simulink model "PIL_NO_RPI"  (R2021a)
settings: Solver=FixedStepAuto  StartTime=0.0  StopTime=50  FixedStep=0.001  RelTol=1e-3  EnableMultiTasking=on
undefined symbols (not defined in the file or in its folder): act_dmp, act_omega, Actuator, Aerodynamics, aMode, Autopilot, c_b_WGS, c_be, c_flat, c_grav, c_h_geop0, c_h_geope, c_pa0, c_pe, c_r0, c_rot, c_rsma, c_Tmp0, d_siB_0, d_siB_max, d_siB_min, dd_siB_max, dd_siB_min, DiscIntNeverNeededParam, e_pa, e_Tmp, fin_maxrate, flag_I_act_switch, flag_I_aero_switch, flag_I_flat, flag_I_gravity_switch, flag_I_rot, hcr, HIL_Data, JMMM_0, JMMM_e, JSPB_e, lat_0, lon_0, Mass_Props, mB_0, mM_0, mM_e, p, pBII_0, phi, pMPB, pNPB, propellant_kg, prp_FBPB, prp_mdot, prp_T, psi, pSPB, q, qEG_0, qIB_0, qIE_0, r, sgc ... (+28)
libraries: simulink x46, simulink_extras x10, aerolibcommonsys x4
(part 5 of 21)

== system PIL_NO_RPI/Non-linear Flight Dynamic Model1/Subsystem1/GRM_Airframe/rb_eom ==
  mot_kin : Inport
  for_mom : Inport  Port=2
  wab : Inport  Port=3
  Bus Creator : BusCreator  Inputs=16
  calc_bus_flight_dyn_bus_entries : Subsystem
  eom_6dof : Subsystem
  flight_dyn : Outport  VectorParamsAs1DForOutWhenUnconnected=off
  wires:
  mot_kin/1 -> calc_bus_flight_dyn_bus_entries/1(mot_kin)
  calc_bus_flight_dyn_bus_entries/1(aBIB) -> Bus Creator/1
  calc_bus_flight_dyn_bus_entries/2(lon) -> Bus Creator/2
  calc_bus_flight_dyn_bus_entries/3(lat) -> Bus Creator/3
  calc_bus_flight_dyn_bus_entries/4(hBE) -> Bus Creator/4
  calc_bus_flight_dyn_bus_entries/5(vBII) -> Bus Creator/5
  calc_bus_flight_dyn_bus_entries/6(qIB) -> Bus Creator/6
  calc_bus_flight_dyn_bus_entries/7(wBIB) -> Bus Creator/7
  calc_bus_flight_dyn_bus_entries/8(d_wBIB) -> Bus Creator/8
  calc_bus_flight_dyn_bus_entries/9(d_vBII) -> Bus Creator/9
  Bus Creator/1 -> flight_dyn/1  "flight_dyn_bus"
  for_mom/1 -> eom_6dof/1(for_mom)
  wab/1 -> eom_6dof/2(wab)
  eom_6dof/1(eom) -> calc_bus_flight_dyn_bus_entries/2(eom)
  calc_bus_flight_dyn_bus_entries/10(pBII) -> Bus Creator/10
  calc_bus_flight_dyn_bus_entries/11(euIB) -> Bus Creator/11
  calc_bus_flight_dyn_bus_entries/12(vBIB) -> Bus Creator/12
  calc_bus_flight_dyn_bus_entries/13(qGB) -> Bus Creator/13
  calc_bus_flight_dyn_bus_entries/14(euGB) -> Bus Creator/14
  calc_bus_flight_dyn_bus_entries/15(euBG) -> Bus Creator/15
  calc_bus_flight_dyn_bus_entries/16(pBLG) -> Bus Creator/16

== system PIL_NO_RPI/Non-linear Flight Dynamic Model1/Subsystem1/GRM_Airframe/stream_flow ==
  flight_dyn : Inport
  motion_kin : Inport  Port=2
  env : Inport  Port=3
  Bus Selector1 : BusSelector  OutputSignals=atm_bus.atm_stat_bus.rho,atm_bus.atm_stat_bus.sos,atm_bus.atm_stat_bus.hBE
  Bus Selector2 : BusSelector  OutputSignals=vBII,pBII,wBIB
  Bus Selector3 : BusSelector  OutputSignals=TIB,wIEE,TIE
  calc_stream_flow : Subsystem
  str_flow : Outport  VectorParamsAs1DForOutWhenUnconnected=off
  wires:
  motion_kin/1 -> Bus Selector3/1
  flight_dyn/1 -> Bus Selector2/1
  env/1 -> Bus Selector1/1
  Bus Selector3/1 -> calc_stream_flow/1(TIB)  "<TIB>"
  Bus Selector3/2 -> calc_stream_flow/2(wIEE)  "<wIEE>"
  Bus Selector3/3 -> calc_stream_flow/3(TIE)  "<TIE>"
  Bus Selector2/1 -> calc_stream_flow/4(VBII)  "<vBII>"
  Bus Selector2/3 -> calc_stream_flow/6(wBIB)  "<wBIB>"
  Bus Selector1/1 -> calc_stream_flow/7(rho)  "<rho>"
  Bus Selector1/2 -> calc_stream_flow/8(sos)  "<sos>"
  Bus Selector1/3 -> calc_stream_flow/9(hBE)  "<hBE>"
  calc_stream_flow/1(str_flow) -> str_flow/1
  Bus Selector2/2 -> calc_stream_flow/5(pBII)  "<pBII>"

== system PIL_NO_RPI/Non-linear Flight Dynamic Model1/Subsystem1/GRM_Airframe/weight_and_balance ==
  env_glb : Inport
  Bus Creator1 : BusCreator  Inputs=3
  Bus Selector2 : BusSelector  OutputSignals=T_sim_glbl,T_sim_lnch
  Subtract : Sum  Inputs=+-
  center_of_gravity : Subsystem
  mass : Subsystem
  mass_uncertainty : Subsystem
  moi : Subsystem
  wab : Outport  VectorParamsAs1DForOutWhenUnconnected=off
  wires:
  Bus Selector2/2 -> Subtract/2  "<T_sim_lnch>"
  Bus Selector2/1 -> Subtract/1  "<T_sim_glbl>"
  env_glb/1 -> Bus Selector2/1
  Bus Creator1/1 -> wab/1  "wab_bus"
  center_of_gravity/1(pBPB) -> moi/1(pBPB), Bus Creator1/2
  moi/1(JBBB) -> Bus Creator1/3
  mass/2(mM) -> moi/2(mM), center_of_gravity/2(mM)
  mass_uncertainty/1(mB) -> center_of_gravity/1(mB), Bus Creator1/1
  mass/1(mB_c) -> mass_uncertainty/1(mB_c)
  Subtract/1 -> mass/1(sim_time_launch)

== system PIL_NO_RPI/Non-linear Flight Dynamic Model2/Extract Relevant States/Assemble_States_Bus1/Rotation Angles to Quaternions ==
  "R1, R2, R3" : Inport  Unit=rad
  1/2 : Gain  Gain=0.5  SaturateOnIntegerOverflow=on  OutDataTypeStr=Inherit: Same as input  ParamDataTypeStr=Inherit: Same as input
  Mux1 : Mux  Inputs=2
  Mux2 : Mux
  q0 : Fcn  Expr=u(4)*u(5)*u(6) + u(1)*u(2)*u(3)
  q1 : Fcn  Expr=u(4)*u(5)*u(3) - u(1)*u(2)*u(6)
  q2 : Fcn  Expr=u(4)*u(2)*u(6) + u(1)*u(5)*u(3)
  q3 : Fcn  Expr=u(1)*u(5)*u(6) - u(4)*u(2)*u(3)
  sincos : Trigonometry  Operator=sincos
  Quat : Outport  Unit=1  InitialOutput=0  VectorParamsAs1DForOutWhenUnconnected=off
  wires:
  q0/1 -> Mux2/1
  Mux2/1 -> Quat/1
  q3/1 -> Mux2/4
  q2/1 -> Mux2/3
  q1/1 -> Mux2/2
  Mux1/1 -> q3/1, q2/1, q1/1, q0/1
  sincos/2 -> Mux1/2
  sincos/1 -> Mux1/1
  1/2/1 -> sincos/1
  "R1, R2, R3"/1 -> 1/2/1

== system PIL_NO_RPI/Non-linear Flight Dynamic Model2/GRM_Airframe/aerodynamics/aerodynamic_via_lookup ==
  pBPB : Inport
  qdynB : Inport  Port=2
  MaB : Inport  Port=3
  alB : Inport  Port=4
  beB : Inport  Port=5
  hBE : Inport  Port=6
  wBIB_star : Inport  Port=7
  afinB : Inport  Port=8
  flag_I_prp : Inport  Port=9
  Bus Creator : BusCreator  Inputs=2
  Demux1 : Demux  Outputs=3
  Demux3 : Demux  Outputs=3
  Gain{,1..4} (5 alike) : Gain  Gain=180/pi
      settings: AttributesFormatString=%<Gain>
  Saturation1 : Saturate  UpperLimit=Aerodynamics.ulim_alpha_deg  LowerLimit=Aerodynamics.llim_alpha_deg
      settings: AttributesFormatString=|
      | %<UpperLimit>
      | %<LowerLimit>
  Saturation4 : Saturate  UpperLimit=Aerodynamics.ulim_beta_deg  LowerLimit=Aerodynamics.llim_beta_deg
      settings: AttributesFormatString=|
      | %<UpperLimit>
      | %<LowerLimit>
  Terminator : Terminator
  Terminator1 : Terminator
  calc_aero_coefficients : Subsystem
  calc_aero_for_mom : Subsystem
  aero_bus : Outport  VectorParamsAs1DForOutWhenUnconnected=off
  wires:
  Gain4/1 -> Saturation4/1
  Gain3/1 -> Saturation1/1
  Saturation4/1 -> calc_aero_coefficients/8(beB_deg)
  Saturation1/1 -> calc_aero_coefficients/7(alB_deg)
  calc_aero_coefficients/6(Cn) -> calc_aero_for_mom/9(Cn)
  calc_aero_coefficients/5(Cm) -> calc_aero_for_mom/8(Cm)
  calc_aero_coefficients/4(Cl) -> calc_aero_for_mom/7(Cl)
  calc_aero_coefficients/3(Cz) -> calc_aero_for_mom/6(Cz)
  calc_aero_coefficients/2(Cy) -> calc_aero_for_mom/5(Cy)
  calc_aero_coefficients/1(Cx) -> calc_aero_for_mom/4(Cx)
  Gain2/1 -> calc_aero_coefficients/3(delr_deg)
  Gain1/1 -> calc_aero_coefficients/2(dele_deg)
  Gain/1 -> calc_aero_coefficients/1(dela_deg)
  Demux3/3 -> Gain2/1  "zeB"
  Demux3/1 -> Gain/1  "xiB"
  Demux3/2 -> Gain1/1  "etB"
  afinB/1 -> Demux3/1
  Demux1/3 -> calc_aero_coefficients/6(rBIB_star_rps)  "rBIB_star_rps"
  Demux1/2 -> calc_aero_coefficients/5(qBIB_star_rps)  "qBIB_star_rps"
  Demux1/1 -> calc_aero_coefficients/4(pBIB_star_rps)  "pBIB_star_rps"
  wBIB_star/1 -> Demux1/1
  beB/1 -> Gain4/1
  alB/1 -> Gain3/1
  qdynB/1 -> calc_aero_for_mom/3(qdynB)
  calc_aero_for_mom/2(MBAB) -> Bus Creator/2
  hBE/1 -> calc_aero_for_mom/1(hBE)
  flag_I_prp/1 -> Terminator/1
  pBPB/1 -> calc_aero_for_mom/2(pBPB)
  Bus Creator/1 -> aero_bus/1  "aero_bus"
  calc_aero_for_mom/1(FBAB) -> Bus Creator/1
  MaB/1 -> Terminator1/1

== system PIL_NO_RPI/Non-linear Flight Dynamic Model2/GRM_Airframe/aerodynamics/logic_base_drag ==
  env_glbl : Inport
  Bus Selector1 : BusSelector  OutputSignals=T_sim_glbl,T_sim_lnch
  Constant : Constant  Value=prp_T(end)
  MATLAB Function : MATLAB Function  TreatAsAtomicUnit=on
  Subtract : Sum  Inputs=+-
  flag_base_drag : Outport  VectorParamsAs1DForOutWhenUnconnected=off
  wires:
  env_glbl/1 -> Bus Selector1/1
  Bus Selector1/2 -> Subtract/2  "<T_sim_lnch>"
  Bus Selector1/1 -> Subtract/1  "<T_sim_glbl>"
  MATLAB Function/1(flag_base_drag) -> flag_base_drag/1  "flag_base_drag"
  Constant/1 -> MATLAB Function/2(t_prp2)
  Subtract/1 -> MATLAB Function/1(u)

== system PIL_NO_RPI/Non-linear Flight Dynamic Model2/GRM_Airframe/environment/WGS84_Gravitation ==
  lon : Inport  PortDimensions=1
  lat : Inport  Port=2  PortDimensions=1
  h : Inport  Port=3  PortDimensions=1
  Assertion : Assertion  AssertionFailFcn="error('WGS84 Gravitationsmodell: Die Werte des Eingangs \"h\" muessen groesser als 0 sein')"
  Assertion1 : Assertion  AssertionFailFcn="error('WGS84 Gravitationsmodell: Die Werte des Eingangs \"Long\" muessen zwischen -180 und +180 liegen')"
  Assertion2 : Assertion  AssertionFailFcn="error('WGS84 Gravitationsmodell: Die Werte des Eingangs \"Lat\" muessen zwischen -90 und +90 liegen')"
  Compare To Constant : simulink/Logic and Bit Operations/Compare To Constant  relop=>=  const=0  OutDataTypeStr=boolean
      settings: SourceProductName=ISim Simulink Block Set
  Interval Test : simulink/Logic and Bit Operations/Interval Test  IntervalClosedRight=on  uplimit=pi  IntervalClosedLeft=on  lowlimit=-pi  OutDataTypeStr=boolean
      settings: SourceProductName=ISim Simulink Block Set
  Interval Test1 : simulink/Logic and Bit Operations/Interval Test  IntervalClosedRight=on  uplimit=pi/2  IntervalClosedLeft=on  lowlimit=-pi/2  OutDataTypeStr=boolean
      settings: SourceProductName=ISim Simulink Block Set
  WGS84_2_ECEF : Subsystem
  WGS84_Gravity_Implementation : MATLAB Function  TreatAsAtomicUnit=on
  gE : Outport  PortDimensions=3  VectorParamsAs1DForOutWhenUnconnected=off
  wires:
  WGS84_Gravity_Implementation/1(gamma_R) -> gE/1  "gE"
  h/1 -> Compare To Constant/1, WGS84_2_ECEF/1(h)  "h"
  lon/1 -> WGS84_2_ECEF/2(lon), Interval Test/1, WGS84_Gravity_Implementation/3(long_rad)  "lon"
  lat/1 -> WGS84_2_ECEF/3(lat), Interval Test1/1, WGS84_Gravity_Implementation/2(lat_rad)  "lat"
  WGS84_2_ECEF/1(pE) -> WGS84_Gravity_Implementation/1(pE)  "pE"
  Compare To Constant/1 -> Assertion/1
  Interval Test/1 -> Assertion1/1
  Interval Test1/1 -> Assertion2/1

== system PIL_NO_RPI/Non-linear Flight Dynamic Model2/GRM_Airframe/environment/atmosphere_static_ISO_2533 ==
  hBE : Inport
  env_glbl : Inport  Port=2
  Bus Creator1 : BusCreator  Inputs=6
  Bus Selector1 : BusSelector  OutputSignals=e_Tmp,e_pa
  Saturation : Saturate  UpperLimit=c_h_geope  LowerLimit=c_h_geop0
      settings: AttributesFormatString=|
      | %<UpperLimit>
      | %<LowerLimit>
  density : Subsystem
  geopot_height : Subsystem  mask{mean_earth_radius=c_r0}
      mask prompts: mean_earth_radius "Mean Earth Radius WGS 84 [m]"
      mask TypeOptions mean_earth_radius: mean_earth_radius/Value
  speed_of_sound : Subsystem
  tmp_and_pressure_ISO_2533 : Subsystem
  atm_stat : Outport  VectorParamsAs1DForOutWhenUnconnected=off
  wires:
  Saturation/1 -> tmp_and_pressure_ISO_2533/1(h_geop), Bus Creator1/2  "h_geop"
  hBE/1 -> geopot_height/1(hBE), Bus Creator1/1
  density/1(rho) -> Bus Creator1/5
  tmp_and_pressure_ISO_2533/2(pa) -> density/2(pa), Bus Creator1/6
  tmp_and_pressure_ISO_2533/1(Tmp) -> density/1(Tmp), Bus Creator1/4, speed_of_sound/1(Tmp)
  Bus Creator1/1 -> atm_stat/1  "atm_stat_bus"
  Bus Selector1/1 -> tmp_and_pressure_ISO_2533/2(e_Tmp)  "<e_Tmp>"
  geopot_height/1(h_geop) -> Saturation/1
  Bus Selector1/2 -> tmp_and_pressure_ISO_2533/3(e_pa)  "<e_pa>"
  env_glbl/1 -> Bus Selector1/1
  speed_of_sound/1(sos) -> Bus Creator1/3

== system PIL_NO_RPI/Non-linear Flight Dynamic Model2/GRM_Airframe/environment/convert_to_local_frame ==
  gE : Inport
  Constant1 : Constant  Value=0
  Dot Product : DotProduct  InputSameDT=on  OutDataTypeStr=Inherit: Inherit via internal rule
  Sqrt : Sqrt  SaturateOnIntegerOverflow=on
  Vector Concatenate : Concatenate  NumInputs=3  Mode=Multidimensional array
  gBG : Outport  VectorParamsAs1DForOutWhenUnconnected=off
  wires:
  Dot Product/1 -> Sqrt/1
  Vector Concatenate/1 -> gBG/1  "gBG"
  Sqrt/1 -> Vector Concatenate/3
  Constant1/1 -> Vector Concatenate/1, Vector Concatenate/2
  gE/1 -> Dot Product/2, Dot Product/1

== system PIL_NO_RPI/Non-linear Flight Dynamic Model2/GRM_Airframe/fin_actuators/Rudder ==
  siB_c : Inport
  tRRR : Inport  Port=2
  Add : Sum  Inputs=+-
  Add1 : Sum  Inputs=+-
  Add2 : Sum  Inputs=+++
  Constant1 : Constant  Value=Actuator.fin1_bias
      settings: AttributesFormatString=%<Value>
  Gain : Gain  Gain=omega^2
  Gain2 : Gain  Gain=2*dmp*omega  Multiplication=Matrix(K*u)
  Gain3 : Gain  Gain=unc_bl
  Gain4 : Gain  Gain=Actuator.fin1_scale
      settings: AttributesFormatString=%<Gain>
  Integrator : Integrator  ExternalReset=either  InitialCondition=d_siB_0
  Integrator1 : Integrator  InitialCondition=siB_0  LimitOutput=on  UpperSaturationLimit=siB_max  LowerSaturationLimit=siB_min  ShowSaturationPort=on
  Limiting_Acceleration : MATLAB Function  TreatAsAtomicUnit=on
  Limiting_Rate : MATLAB Function  TreatAsAtomicUnit=on
  Saturation : Saturate  UpperLimit=siB_max  LowerLimit=siB_min
  Saturation1 : Saturate  UpperLimit=siB_max  LowerLimit=siB_min
  Sign : Signum
  siB : Outport  VectorParamsAs1DForOutWhenUnconnected=off
  d_siB : Outport  Port=2  VectorParamsAs1DForOutWhenUnconnected=off
  dd_siB : Outport  Port=3  VectorParamsAs1DForOutWhenUnconnected=off
  wires:
  [siB] -> Limiting_Rate/1(siB)
  [siB] -> Limiting_Acceleration/1(siB)
  [d_siB] -> Limiting_Acceleration/2(d_siB)
  siB_c/1 -> Saturation/1  "siB_c"
  Constant1/1 -> Add2/1
  Add2/1 -> Saturation1/1
  Saturation/1 -> Add/1
  Integrator/1 -> Gain2/1, Limiting_Rate/2(d_siB)  "d_siB"
  Limiting_Rate/1(d_siB_l) -> Integrator1/1, [d_siB], d_siB/1  "d_siB_l"
  Limiting_Acceleration/1(dd_siB_l) -> dd_siB/1, Integrator/1  "dd_siB_l"
  Add/1 -> Gain/1
  Gain/1 -> Add1/1
  Gain2/1 -> Add1/2
  Add1/1 -> Limiting_Acceleration/3(dd_siB)  "dd_siB"
  Integrator1/1 -> Add/2, Gain4/1  "siB"
  tRRR/1 -> Sign/1  "tRRR"
  Sign/1 -> Gain3/1
  Gain3/1 -> Add2/3
  Gain4/1 -> Add2/2
  Integrator1/2 -> Integrator/2  "sat"
  Saturation1/1 -> [siB], siB/1  "siB"

== system PIL_NO_RPI/Non-linear Flight Dynamic Model2/GRM_Airframe/fin_actuators/Rudder1 ==
  siB_c : Inport
  tRRR : Inport  Port=2
  Add : Sum  Inputs=+-
  Add1 : Sum  Inputs=+-
  Add3 : Sum  Inputs=+++
  Constant1 : Constant  Value=Actuator.fin2_bias
      settings: AttributesFormatString=%<Value>
  Gain : Gain  Gain=omega^2
  Gain2 : Gain  Gain=2*dmp*omega  Multiplication=Matrix(K*u)
  Gain3 : Gain  Gain=unc_bl
  Gain4 : Gain  Gain=Actuator.fin2_scale
      settings: AttributesFormatString=%<Gain>
  Integrator : Integrator  ExternalReset=either  InitialCondition=d_siB_0
  Integrator1 : Integrator  InitialCondition=siB_0  LimitOutput=on  UpperSaturationLimit=siB_max  LowerSaturationLimit=siB_min  ShowSaturationPort=on
  Limiting_Acceleration : MATLAB Function  TreatAsAtomicUnit=on
  Limiting_Rate : MATLAB Function  TreatAsAtomicUnit=on
  Saturation : Saturate  UpperLimit=siB_max  LowerLimit=siB_min
  Saturation1 : Saturate  UpperLimit=siB_max  LowerLimit=siB_min
  Sign : Signum
  siB : Outport  VectorParamsAs1DForOutWhenUnconnected=off
  d_siB : Outport  Port=2  VectorParamsAs1DForOutWhenUnconnected=off
  dd_siB : Outport  Port=3  VectorParamsAs1DForOutWhenUnconnected=off
  wires:
  Gain4/1 -> Add3/2
  Constant1/1 -> Add3/1
  [siB] -> Limiting_Rate/1(siB)
  [siB] -> Limiting_Acceleration/1(siB)
  [d_siB] -> Limiting_Acceleration/2(d_siB)
  siB_c/1 -> Saturation/1  "siB_c"
  Add3/1 -> Saturation1/1
  Saturation/1 -> Add/1
  Integrator/1 -> Gain2/1, Limiting_Rate/2(d_siB)  "d_siB"
  Limiting_Rate/1(d_siB_l) -> Integrator1/1, [d_siB], d_siB/1  "d_siB_l"
  Limiting_Acceleration/1(dd_siB_l) -> dd_siB/1, Integrator/1  "dd_siB_l"
  Add/1 -> Gain/1
  Gain/1 -> Add1/1
  Gain2/1 -> Add1/2
  Add1/1 -> Limiting_Acceleration/3(dd_siB)  "dd_siB"
  Integrator1/1 -> Gain4/1, Add/2  "siB"
  tRRR/1 -> Sign/1  "tRRR"
  Sign/1 -> Gain3/1
  Gain3/1 -> Add3/3
  Integrator1/2 -> Integrator/2  "sat"
  Saturation1/1 -> [siB], siB/1  "siB"

== system PIL_NO_RPI/Non-linear Flight Dynamic Model2/GRM_Airframe/fin_actuators/Rudder2 ==
  siB_c : Inport
  tRRR : Inport  Port=2
  Add : Sum  Inputs=+-
  Add1 : Sum  Inputs=+-
  Add3 : Sum  Inputs=+++
  Constant1 : Constant  Value=Actuator.fin3_bias
      settings: AttributesFormatString=%<Value>
  Gain : Gain  Gain=omega^2
  Gain2 : Gain  Gain=2*dmp*omega  Multiplication=Matrix(K*u)
  Gain3 : Gain  Gain=unc_bl
  Gain4 : Gain  Gain=Actuator.fin3_scale
      settings: AttributesFormatString=%<Gain>
  Integrator : Integrator  ExternalReset=either  InitialCondition=d_siB_0
  Integrator1 : Integrator  InitialCondition=siB_0  LimitOutput=on  UpperSaturationLimit=siB_max  LowerSaturationLimit=siB_min  ShowSaturationPort=on
  Limiting_Acceleration : MATLAB Function  TreatAsAtomicUnit=on
  Limiting_Rate : MATLAB Function  TreatAsAtomicUnit=on
  Saturation : Saturate  UpperLimit=siB_max  LowerLimit=siB_min
  Saturation1 : Saturate  UpperLimit=siB_max  LowerLimit=siB_min
  Sign : Signum
  siB : Outport  VectorParamsAs1DForOutWhenUnconnected=off
  d_siB : Outport  Port=2  VectorParamsAs1DForOutWhenUnconnected=off
  dd_siB : Outport  Port=3  VectorParamsAs1DForOutWhenUnconnected=off
  wires:
  Gain4/1 -> Add3/2
  Constant1/1 -> Add3/1
  [siB] -> Limiting_Rate/1(siB)
  [siB] -> Limiting_Acceleration/1(siB)
  [d_siB] -> Limiting_Acceleration/2(d_siB)
  siB_c/1 -> Saturation/1  "siB_c"
  Add3/1 -> Saturation1/1
  Saturation/1 -> Add/1
  Integrator/1 -> Gain2/1, Limiting_Rate/2(d_siB)  "d_siB"
  Limiting_Rate/1(d_siB_l) -> Integrator1/1, [d_siB], d_siB/1  "d_siB_l"
  Limiting_Acceleration/1(dd_siB_l) -> dd_siB/1, Integrator/1  "dd_siB_l"
  Add/1 -> Gain/1
  Gain/1 -> Add1/1
  Gain2/1 -> Add1/2
  Add1/1 -> Limiting_Acceleration/3(dd_siB)  "dd_siB"
  Integrator1/1 -> Add/2, Gain4/1  "siB"
  tRRR/1 -> Sign/1  "tRRR"
  Sign/1 -> Gain3/1
  Gain3/1 -> Add3/3
  Integrator1/2 -> Integrator/2  "sat"
  Saturation1/1 -> [siB], siB/1  "siB"

== system PIL_NO_RPI/Non-linear Flight Dynamic Model2/GRM_Airframe/fin_actuators/Rudder3 ==
  siB_c : Inport
  tRRR : Inport  Port=2
  Add : Sum  Inputs=+-
  Add1 : Sum  Inputs=+-
  Add3 : Sum  Inputs=+++
  Constant1 : Constant  Value=Actuator.fin4_bias
      settings: AttributesFormatString=%<Value>
  Gain : Gain  Gain=omega^2
  Gain2 : Gain  Gain=2*dmp*omega  Multiplication=Matrix(K*u)
  Gain3 : Gain  Gain=unc_bl
  Gain4 : Gain  Gain=Actuator.fin4_scale
      settings: AttributesFormatString=%<Gain>
  Integrator : Integrator  ExternalReset=either  InitialCondition=d_siB_0
  Integrator1 : Integrator  InitialCondition=siB_0  LimitOutput=on  UpperSaturationLimit=siB_max  LowerSaturationLimit=siB_min  ShowSaturationPort=on
  Limiting_Acceleration : MATLAB Function  TreatAsAtomicUnit=on
  Limiting_Rate : MATLAB Function  TreatAsAtomicUnit=on
  Saturation : Saturate  UpperLimit=siB_max  LowerLimit=siB_min
  Saturation1 : Saturate  UpperLimit=siB_max  LowerLimit=siB_min
  Sign : Signum
  siB : Outport  VectorParamsAs1DForOutWhenUnconnected=off
  d_siB : Outport  Port=2  VectorParamsAs1DForOutWhenUnconnected=off
  dd_siB : Outport  Port=3  VectorParamsAs1DForOutWhenUnconnected=off
  wires:
  Gain4/1 -> Add3/2
  Constant1/1 -> Add3/1
  [siB] -> Limiting_Rate/1(siB)
  [siB] -> Limiting_Acceleration/1(siB)
  [d_siB] -> Limiting_Acceleration/2(d_siB)
  siB_c/1 -> Saturation/1  "siB_c"
  Add3/1 -> Saturation1/1
  Saturation/1 -> Add/1
  Integrator/1 -> Gain2/1, Limiting_Rate/2(d_siB)  "d_siB"
  Limiting_Rate/1(d_siB_l) -> Integrator1/1, [d_siB], d_siB/1  "d_siB_l"
  Limiting_Acceleration/1(dd_siB_l) -> dd_siB/1, Integrator/1  "dd_siB_l"
  Add/1 -> Gain/1
  Gain/1 -> Add1/1
  Gain2/1 -> Add1/2
  Add1/1 -> Limiting_Acceleration/3(dd_siB)  "dd_siB"
  Integrator1/1 -> Add/2, Gain4/1  "siB"
  tRRR/1 -> Sign/1  "tRRR"
  Sign/1 -> Gain3/1
  Gain3/1 -> Add3/3
  Integrator1/2 -> Integrator/2  "sat"
  Saturation1/1 -> [siB], siB/1  "siB"

== system PIL_NO_RPI/Non-linear Flight Dynamic Model2/GRM_Airframe/fin_actuators/control_allocation ==
  siB : Inport
  d_siB : Inport  Port=2
  dd_siB : Inport  Port=3
  Constant8 : Constant  Value=Tr3r4
  Product : Product  Multiplication=Matrix(*)
  Product1 : Product  Multiplication=Matrix(*)
  Product2 : Product  Multiplication=Matrix(*)
  Tr3r4 : Outport  VectorParamsAs1DForOutWhenUnconnected=off
  finB : Outport  Port=2  VectorParamsAs1DForOutWhenUnconnected=off
  d_finB : Outport  Port=3  VectorParamsAs1DForOutWhenUnconnected=off
  dd_finB : Outport  Port=4  VectorParamsAs1DForOutWhenUnconnected=off
  wires:
  Product2/1 -> dd_finB/1  "dd_afinB"
  dd_siB/1 -> Product2/2
  Product1/1 -> d_finB/1  "d_afinB"
  d_siB/1 -> Product1/2
  siB/1 -> Product/2
  Constant8/1 -> Product/1, Product1/1, Product2/1, Tr3r4/1  "Tr3r4"
  Product/1 -> finB/1  "afinB"

== system PIL_NO_RPI/Non-linear Flight Dynamic Model2/GRM_Airframe/gravity/launch_rail ==
  gBG_c : Inport
  hBE : Inport  Port=2
  Constant1 : Constant  Value=flag_I_gravity_switch
  Constant3 : Constant  Value=0
  Subtract : Sum  Inputs=++-
  Switch : Switch  Criteria=u2 > Threshold  Threshold=0.05
  Vector Concatenate : Concatenate  NumInputs=3
  initial_altitude : Subsystem
  gBG : Outport  VectorParamsAs1DForOutWhenUnconnected=off
  wires:
  initial_altitude/1(hBE_0) -> Subtract/3
  gBG_c/1 -> Switch/1
  Vector Concatenate/1 -> Switch/3
  Switch/1 -> gBG/1  "gBG"
  Constant3/1 -> Vector Concatenate/3, Vector Concatenate/2, Vector Concatenate/1
  Subtract/1 -> Switch/2
  hBE/1 -> Subtract/1
  Constant1/1 -> Subtract/2

== system PIL_NO_RPI/Non-linear Flight Dynamic Model2/GRM_Airframe/motion_kinematics/calc_motion_kinematics ==
  lat : Inport
  lon : Inport  Port=2
  qIB : Inport  Port=3
  calc_transformation_matrix : Subsystem
  earth_rotation : Subsystem
  wIEE : Outport  VectorParamsAs1DForOutWhenUnconnected=off
  TIE : Outport  Port=2  VectorParamsAs1DForOutWhenUnconnected=off
  TEB : Outport  Port=3  VectorParamsAs1DForOutWhenUnconnected=off
  TGB : Outport  Port=4  VectorParamsAs1DForOutWhenUnconnected=off
  TEG : Outport  Port=5  VectorParamsAs1DForOutWhenUnconnected=off
  wEGG : Outport  Port=6  VectorParamsAs1DForOutWhenUnconnected=off
  TIB : Outport  Port=7  VectorParamsAs1DForOutWhenUnconnected=off
  wires:
  calc_transformation_matrix/3(TIB) -> TIB/1
  calc_transformation_matrix/2(TGB) -> TGB/1
  calc_transformation_matrix/1(TEB) -> TEB/1
  qIB/1 -> calc_transformation_matrix/3(qIB)
  earth_rotation/4(qEG) -> calc_transformation_matrix/2(qEG)
  earth_rotation/3(qIE) -> calc_transformation_matrix/1(qIE)
  lat/1 -> earth_rotation/1(lat)
  lon/1 -> earth_rotation/2(lon)
  earth_rotation/6(wEGG) -> wEGG/1
  earth_rotation/5(TEG) -> TEG/1
  earth_rotation/2(TIE) -> TIE/1
  earth_rotation/1(wIEE) -> wIEE/1

== system PIL_NO_RPI/Non-linear Flight Dynamic Model2/GRM_Airframe/propulsion/prp_look_up ==
  env_glbl_bus : Inport
  Bus Selector1 : BusSelector  OutputSignals=T_sim_glbl,T_sim_lnch
  Constant : Constant  Value=0
  Constant1 : Constant  Value=0
  Saturation : Saturate  UpperLimit=prp_T(end)  LowerLimit=0
      settings: AttributesFormatString=|
      | %<UpperLimit>
      | %<LowerLimit>
  Subtract : Sum  Inputs=+-
  Switch : Switch  Criteria=u2 > Threshold
  Switch1 : Switch  Criteria=u2 > Threshold
  Vector Concatenate : Concatenate  NumInputs=3
  thrust_lookup : Lookup_n-D  NumberOfTableDimensions=1  BreakpointsForDimension1=prp_T  Table=prp_FBPB  ExtrapMethod=Clip  UseLastTableValue=on  InternalRulePriority=Speed  RndMeth=Simplest  InputSameDT=on
  FBPM : Outport  VectorParamsAs1DForOutWhenUnconnected=off
  wires:
  Switch1/1 -> Vector Concatenate/1  "a_FBPM"
  Constant1/1 -> Vector Concatenate/2, Vector Concatenate/3
  Vector Concatenate/1 -> FBPM/1  "FBPM"
  Saturation/1 -> thrust_lookup/1
  Subtract/1 -> Switch/2, Switch/1
  Constant/1 -> Switch/3
  env_glbl_bus/1 -> Bus Selector1/1
  Bus Selector1/1 -> Subtract/1  "<T_sim_glbl>"
  thrust_lookup/1 -> Switch1/1
  Switch/1 -> Switch1/3, Switch1/2, Saturation/1
  Bus Selector1/2 -> Subtract/2  "<T_sim_lnch>"

== system PIL_NO_RPI/Non-linear Flight Dynamic Model2/GRM_Airframe/propulsion/prp_uncertainty ==
  FBPM : Inport
  wab : Inport  Port=2
  3_rot_mat : Subsystem  mask(Rotation um 1, 2 oder 3 Achsen){rot_1=Rotation um z-Achse, rot_2=Rotation um y-Achse, rot_3=Rotation um x-Achse}
      mask prompts: rot_1 "1. Rotation"; rot_2 "2. Rotation"; rot_3 "3. Rotation"
      mask help:
      | Dieser Block liefert die Rotationsmatrix T12 für den Fall zurück, dass sich das Ziel-Koordinatensystem (1) durch Drehungen um 1, 2 oder 3 Achsen gegenüber dem Ausgangskoordinatensystem (2) beschreiben lässt (passive Drehung).
      |
      | Die Anzahl der Rotation sowie die Reihenfolge ist frei einstellbar.
      |
      | Die Rotationswinkel haben die Einheit [rad].
      mask TypeOptions rot_1: Rotation um x-Achse | Rotation um y-Achse | Rotation um z-Achse
      mask TypeOptions rot_2: Rotation um x-Achse | Rotation um y-Achse | Rotation um z-Achse
      mask TypeOptions rot_3: Rotation um x-Achse | Rotation um y-Achse | Rotation um z-Achse
  Bus Selector : BusSelector  OutputSignals=pBPB
  Product : Product  Multiplication=Matrix(*)
  Product1 : Product
  Subtract : Sum  Inputs=+-
  Thrust_rot_z : Constant  Value=unc_prp_z
  cross_product : Subsystem
      mask help: cross product r3 = r1 x r2
      mask Help:
      | Name:
      | 
      |     cross_product
      | 
      | Description:
      | 
      |     This block implements the cross product r3 = r1 x r2.
      | 
      | Inputs  [size] [data type] [unit]:
      | 
      |     vector 1  [3] [double] [-]
      |     vector 2  [3] [double] [-]
      | 
      | Outputs  [size] [data type] [unit]:
      | 
      |     resulting vector  [3] [double] [-]
      mask Display: disp(' r3 = r1 x r2')
  pNPB : Constant  Value=pNPB
  thrust_rot_x : Constant  Value=unc_prp_x
  thrust_rot_y : Constant  Value=unc_prp_y
  uncert_thrust : Constant  Value=unc_prp_scale
  FBPB : Outport  VectorParamsAs1DForOutWhenUnconnected=off
  MBPB : Outport  Port=2  VectorParamsAs1DForOutWhenUnconnected=off
  wires:
  Subtract/1 -> cross_product/1(r1)
  pNPB/1 -> Subtract/2
  Product1/1 -> Product/2
  uncert_thrust/1 -> Product1/2
  Bus Selector/1 -> Subtract/1  "<pBPB>"
  wab/1 -> Bus Selector/1
  cross_product/1(r1_x_r2) -> MBPB/1  "MBPB"
  thrust_rot_y/1 -> 3_rot_mat/2(wi2)
  3_rot_mat/1(T12) -> Product/1
  FBPM/1 -> Product1/1
  Product/1 -> FBPB/1, cross_product/2(r2)  "FBPB"
  thrust_rot_x/1 -> 3_rot_mat/3(wi3)
  Thrust_rot_z/1 -> 3_rot_mat/1(wi1)

== system PIL_NO_RPI/Non-linear Flight Dynamic Model2/GRM_Airframe/rb_eom/calc_bus_flight_dyn_bus_entries ==
  mot_kin : Inport
  eom : Inport  Port=2
  Bus Selector : BusSelector  OutputSignals=pBII,vBII,qIB,wBIB,d_wBIB,d_vBII
  Bus Selector1 : BusSelector  OutputSignals=pBII
  Bus Selector3 : BusSelector  OutputSignals=TGB,TIB,TIE
  Constant : Constant  Value=pBII_0
      settings: AttributesFormatString=%<Value>
  Gain : Gain  Gain=-1
  Math Function : Math  Operator=transpose  SignedPower=on  SaturateOnIntegerOverflow=on
  Product{,1..3} (4 alike) : Product  Multiplication=Matrix(*)
  Subsystem2 : Subsystem
  Sum : Sum  Inputs=+-
  eom D1 : InportShadow  Port=2
  q12_from_T12 : Subsystem
      mask help: Transforms a Direction Cosine Matrix into a Quaternion
      mask Help:
      | Name:
      | 
      |     q12_from_T12
      | 
      | Description:
      | 
      |     This block implements the transformation of a direction cosine matrix DCM
      |      into the corresponding quaternion.
      | 
      | Inputs  [size] [data type] [unit]:
      | 
      |     direction cosine matrix T12  [3x3] [double] [-]
      | 
      | Outputs  [size] [data type] [unit]:
      | 
      |     quaternion q12  [4] [double] [-]
      mask Display:
      | %port_label('input', 1, 'T12')
      | %port_label('output', 1, 'q12')
      | disp('DCM \rightarrow q','texmode','on')
  quaternion_to_euler_angles : Subsystem
      mask help: transforms quaternions to Euler angles (roll, pitch, yaw)
      mask Help:
      | Name:
      | 
      |     quaternion_to_euler_angles
      | 
      | Description:
      | 
      |     This block implements the transformation of a quaternion into the
      |     corresponding Euler angles (zyx-sequence, roll, pitch, yaw).
      | 
      | Inputs  [size] [data type] [unit]:
      | 
      |     quaternion  [4] [double] [-]
      | 
      | Outputs  [size] [data type] [unit]:
      | 
      |     roll angle phi  [1] [double] [rad]
      |     pitch angle theta  [1] [double] [rad]
      |     yaw angle psi  [1] [double] [rad]
      mask Display:
      | %disp (' q --> (Phi,Theta,Psi) [rad]')
      | disp('q \rightarrow eu(\Phi;\Theta;\Psi)','texmode','on')
  quaternion_to_euler_angles1 : Subsystem
      mask help: transforms quaternions to Euler angles (roll, pitch, yaw)
      mask Help:
      | Name:
      | 
      |     quaternion_to_euler_angles
      | 
      | Description:
      | 
      |     This block implements the transformation of a quaternion into the
      |     corresponding Euler angles (zyx-sequence, roll, pitch, yaw).
      | 
      | Inputs  [size] [data type] [unit]:
      | 
      |     quaternion  [4] [double] [-]
      | 
      | Outputs  [size] [data type] [unit]:
      | 
      |     roll angle phi  [1] [double] [rad]
      |     pitch angle theta  [1] [double] [rad]
      |     yaw angle psi  [1] [double] [rad]
      mask Display:
      | %disp (' q --> (Phi,Theta,Psi) [rad]')
      | disp('q \rightarrow eu(\Phi;\Theta;\Psi)','texmode','on')
  aBIB : Outport  VectorParamsAs1DForOutWhenUnconnected=off
  lon : Outport  Port=2  VectorParamsAs1DForOutWhenUnconnected=off
  lat : Outport  Port=3  VectorParamsAs1DForOutWhenUnconnected=off
  hBE : Outport  Port=4  VectorParamsAs1DForOutWhenUnconnected=off
  vBII : Outport  Port=5  VectorParamsAs1DForOutWhenUnconnected=off
  qIB : Outport  Port=6  VectorParamsAs1DForOutWhenUnconnected=off
  wBIB : Outport  Port=7  VectorParamsAs1DForOutWhenUnconnected=off
  d_wBIB : Outport  Port=8  VectorParamsAs1DForOutWhenUnconnected=off
  d_vBII : Outport  Port=9  VectorParamsAs1DForOutWhenUnconnected=off
  pBII : Outport  Port=10  VectorParamsAs1DForOutWhenUnconnected=off
  euIB : Outport  Port=11  VectorParamsAs1DForOutWhenUnconnected=off
  vBIB : Outport  Port=12  VectorParamsAs1DForOutWhenUnconnected=off
  qGB : Outport  Port=13  VectorParamsAs1DForOutWhenUnconnected=off
  euGB : Outport  Port=14  VectorParamsAs1DForOutWhenUnconnected=off
  euBG : Outport  Port=15  VectorParamsAs1DForOutWhenUnconnected=off
  pBLG : Outport  Port=16  VectorParamsAs1DForOutWhenUnconnected=off
  wires:
  Product3/1 -> pBLG/1  "pBLG"
  Product2/1 -> Product3/1  "TGI"
  [TBI] -> Product2/2
  [TGB] -> Product2/1
  Sum/1 -> Product3/2  "pBLI"
  Constant/1 -> Sum/2
  Bus Selector1/1 -> Sum/1  "<pBII>"
  eom D1/1 -> Bus Selector1/1
  Gain/1 -> euBG/1  "euBG"
  quaternion_to_euler_angles1/1(eulx) -> Gain/1, euGB/1  "euGB"
  q12_from_T12/1(q12) -> qGB/1, quaternion_to_euler_angles1/1(q)  "qGB"
  Bus Selector3/1 -> q12_from_T12/1(T12), [TGB]  "<TGB>"
  Product1/1 -> vBIB/1  "vBIB"
  quaternion_to_euler_angles/1(eulx) -> euIB/1  "euIB"
  Bus Selector/5 -> d_wBIB/1  "<d_wBIB>"
  Bus Selector/4 -> wBIB/1  "<wBIB>"
  Bus Selector/3 -> qIB/1, quaternion_to_euler_angles/1(q)  "<qIB>"
  Bus Selector/2 -> vBII/1, Product1/2  "<vBII>"
  Subsystem2/3(hBE) -> hBE/1  "hBE"
  Subsystem2/2(lat) -> lat/1
  Subsystem2/1(lon) -> lon/1
  Product/1 -> aBIB/1  "aBIB"
  Bus Selector/6 -> d_vBII/1, Product/2  "<d_vBII>"
  Bus Selector3/2 -> Math Function/1  "<TIB>"
  Math Function/1 -> Product/1, Product1/1, [TBI]  "TBI"
  eom/1 -> Bus Selector/1
  Bus Selector3/3 -> Subsystem2/1(TIE)  "<TIE>"
  mot_kin/1 -> Bus Selector3/1
  Bus Selector/1 -> Subsystem2/2(pBII), pBII/1  "<pBII>"

== system PIL_NO_RPI/Non-linear Flight Dynamic Model2/GRM_Airframe/rb_eom/eom_6dof ==
  for_mom : Inport
  wab : Inport  Port=2
  Bus Selector1 : BusSelector  OutputSignals=mB,JBBB
  Bus Selector2 : BusSelector  OutputSignals=FBTB,MBTB
  Constant : Constant  Value=[pBII_0; vBII_0; qIB_0; wBIB_0]
  Constant9 : Constant  Value=[0 0 0; 0 0 0; 0 0 0]
  Rigid_Body_EOM_6_DOF : Subsystem  mask{flag_Kraft=FBTB}
      mask prompts: flag_Kraft "Input Kraftvektor"
      mask help:
      | 6DOF-Bewegungsgleichungen im ECI-System mit
      | zeitvariantem Massenträgheitsmoment.
      |
      | Modell Varianten:
      | - Koordinatensystem des Kraftvektor:
      |      FBTI : Inertial System I
      |      FBTB : Körperfestes System B
      mask init:
      | switch flag_Kraft
      |     case 1
      |         port_label_kraft = 'FBTI';
      |     case 2
      |         port_label_kraft = 'FBTB';
      | end
      mask TypeOptions flag_Kraft: FBTI | FBTB
      mask DialogControl Container4 Prompt: Modell Einstellungen
      mask Display:
      | port_label ('input',1,port_label_kraft )
      | port_label ('input',2,'MBTB' )
      | port_label ('input',3,'mB' )
      | port_label ('input',4,'x0' )
      | port_label ('input',5,'JBB' )
      | port_label ('input',6,'d_JBB' )
      | port_label ('output',1,'rb_eom' )
  eom : Outport  VectorParamsAs1DForOutWhenUnconnected=off
  wires:
  wab/1 -> Bus Selector1/1
  Bus Selector1/1 -> Rigid_Body_EOM_6_DOF/3(mB)  "<mB>"
  Constant/1 -> Rigid_Body_EOM_6_DOF/4(x0)
  for_mom/1 -> Bus Selector2/1
  Bus Selector1/2 -> Rigid_Body_EOM_6_DOF/5(JBB)  "<JBBB>"
  Constant9/1 -> Rigid_Body_EOM_6_DOF/6(d_JBB)
  Rigid_Body_EOM_6_DOF/1(rb_eom) -> eom/1
  Bus Selector2/1 -> Rigid_Body_EOM_6_DOF/1(FBTX)  "<FBTB>"
  Bus Selector2/2 -> Rigid_Body_EOM_6_DOF/2(MBTB)  "<MBTB>"

== system PIL_NO_RPI/Non-linear Flight Dynamic Model2/GRM_Airframe/stream_flow/calc_stream_flow ==
  TIB : Inport
  wIEE : Inport  Port=2
  TIE : Inport  Port=3
  VBII : Inport  Port=4
  pBII : Inport  Port=5
  wBIB : Inport  Port=6
  rho : Inport  Port=7
  sos : Inport  Port=8
  hBE : Inport  Port=9
  Bus Creator : BusCreator  Inputs=9
  Math Function : Math  Operator=transpose  SignedPower=on  SaturateOnIntegerOverflow=on
  Product : Product  Multiplication=Matrix(*)
  Subsystem1 : Subsystem
  velocity_vector_transformation : Subsystem
  str_flow : Outport  VectorParamsAs1DForOutWhenUnconnected=off
  wires:
  pBII/1 -> velocity_vector_transformation/4(pBII)
  TIB/1 -> Math Function/1
  rho/1 -> Subsystem1/3(rho)
  sos/1 -> Subsystem1/4(sos)
  hBE/1 -> Bus Creator/9
  wBIB/1 -> Subsystem1/2(wBIB)
  Bus Creator/1 -> str_flow/1  "str_flow_bus"
  wIEE/1 -> velocity_vector_transformation/1(wIEE)
  Subsystem1/1(al) -> Bus Creator/1  "alB"
  Subsystem1/7(th) -> Bus Creator/7  "inB"
  velocity_vector_transformation/1(vBEI) -> Product/2
  Subsystem1/3(qdynB) -> Bus Creator/3
  TIE/1 -> velocity_vector_transformation/2(TIE)
  Subsystem1/6(wBIB_star) -> Bus Creator/6
  Product/1 -> Subsystem1/1(vBEB)  "vBEB"
  Subsystem1/5(a_vB) -> Bus Creator/5
  VBII/1 -> velocity_vector_transformation/3(vBII)
  Subsystem1/8(fi) -> Bus Creator/8  "fiB"
  Subsystem1/2(be) -> Bus Creator/2  "beB"
  Math Function/1 -> Product/1  "TBI"
  Subsystem1/4(MaB) -> Bus Creator/4

== system PIL_NO_RPI/Non-linear Flight Dynamic Model2/GRM_Airframe/weight_and_balance/center_of_gravity ==
  mB : Inport
  mM : Inport  Port=2
  1-D Lookup Table : Lookup_n-D  NumberOfTableDimensions=1  BreakpointsForDimension1=Mass_Props.propellant_bkpts  Table=Mass_Props.CGx_m_tbl  ExtrapMethod=Clip  UseLastTableValue=on  InternalRulePriority=Speed  RndMeth=Simplest  InputSameDT=on
      settings: AttributesFormatString=|
      | %<Table>
      | %<BreakpointsForDimension1>
  1-D Lookup Table3 : Lookup_n-D  NumberOfTableDimensions=1  BreakpointsForDimension1=Mass_Props.propellant_bkpts  Table=Mass_Props.CGy_m_tbl  ExtrapMethod=Clip  UseLastTableValue=on  InternalRulePriority=Speed  RndMeth=Simplest  InputSameDT=on
      settings: AttributesFormatString=|
      | %<Table>
      | %<BreakpointsForDimension1>
  1-D Lookup Table6 : Lookup_n-D  NumberOfTableDimensions=1  BreakpointsForDimension1=Mass_Props.propellant_bkpts  Table=Mass_Props.CGz_m_tbl  ExtrapMethod=Clip  UseLastTableValue=on  InternalRulePriority=Speed  RndMeth=Simplest  InputSameDT=on
      settings: AttributesFormatString=|
      | %<Table>
      | %<BreakpointsForDimension1>
  Add6 : Sum
  Add7 : Sum
  Add8 : Sum
  Constant10 : Constant  Value=unc_cg_x
  Constant11 : Constant  Value=unc_cg_y
  Constant12 : Constant  Value=unc_cg_z
  Terminator1 : Terminator
  Vector Concatenate1 : Concatenate  NumInputs=3
  mM D2 : InportShadow  Port=2
  mM D3 : InportShadow  Port=2
  pBPB : Outport  VectorParamsAs1DForOutWhenUnconnected=off
  wires:
  mB/1 -> Terminator1/1
  Add8/1 -> Vector Concatenate1/3
  Constant12/1 -> Add8/2
  Add7/1 -> Vector Concatenate1/2
  Constant11/1 -> Add7/2
  Constant10/1 -> Add6/2
  Add6/1 -> Vector Concatenate1/1
  mM D3/1 -> 1-D Lookup Table6/1
  mM D2/1 -> 1-D Lookup Table3/1
  mM/1 -> 1-D Lookup Table/1
  1-D Lookup Table/1 -> Add6/1
  Vector Concatenate1/1 -> pBPB/1  "pBPB"
  1-D Lookup Table3/1 -> Add7/1
  1-D Lookup Table6/1 -> Add8/1

== system PIL_NO_RPI/Non-linear Flight Dynamic Model2/GRM_Airframe/weight_and_balance/mass ==
  sim_time_launch : Inport
  1-D Lookup Table2 : Lookup_n-D  NumberOfTableDimensions=1  BreakpointsForDimension1=prp_T  Table=prp_mdot  ExtrapMethod=Clip  DiagnosticForOutOfRangeInput=Warning  UseLastTableValue=on  InternalRulePriority=Speed  RndMeth=Simplest  InputSameDT=on
  Constant : Constant  Value=0
  Constant1 : Constant  Value=mB_0
  Constant2 : Constant  Value=propellant_kg
      settings: AttributesFormatString=%<Value>
  Gain : Gain  Gain=-1
  Integrator1 : Integrator  InitialConditionSource=external
  Saturation : Saturate  UpperLimit=prp_T(end)  LowerLimit=0
      settings: AttributesFormatString=|
      | %<UpperLimit>
      | %<LowerLimit>
  Subtract1 : Sum
  Switch : Switch  Criteria=u2 > Threshold
  Switch1 : Switch  Criteria=u2 > Threshold
  mB_c : Outport  VectorParamsAs1DForOutWhenUnconnected=off
  mM : Outport  Port=2  VectorParamsAs1DForOutWhenUnconnected=off
  wires:
  Integrator1/1 -> Switch1/1  "propellant_remaining_kg"
  Gain/1 -> Integrator1/1
  1-D Lookup Table2/1 -> Gain/1  "mdot_kgps"
  Constant2/1 -> Integrator1/2
  Switch1/1 -> Subtract1/2, mM/1  "mM"
  Saturation/1 -> 1-D Lookup Table2/1
  sim_time_launch/1 -> Switch/2, Switch/1
  Constant/1 -> Switch/3
  Switch/1 -> Saturation/1, Switch1/3, Switch1/2
  Subtract1/1 -> mB_c/1  "mB_c"
  Constant1/1 -> Subtract1/1

== system PIL_NO_RPI/Non-linear Flight Dynamic Model2/GRM_Airframe/weight_and_balance/mass_uncertainty ==
  mB_c : Inport
  Add : Sum
  Constant : Constant  Value=unc_mB_bl
  Constant1 : Constant  Value=unc_mB_scale
  Product : Product
  mB : Outport  VectorParamsAs1DForOutWhenUnconnected=off
  wires:
  Product/1 -> Add/2
  Constant1/1 -> Product/2
  Add/1 -> mB/1  "mB"
  mB_c/1 -> Product/1
  Constant/1 -> Add/1

== system PIL_NO_RPI/Non-linear Flight Dynamic Model2/GRM_Airframe/weight_and_balance/moi ==
  pBPB : Inport
  mM : Inport  Port=2
  1-D Lookup Table : Lookup_n-D  NumberOfTableDimensions=1  BreakpointsForDimension1=Mass_Props.propellant_bkpts  Table=Mass_Props.Ixx_tbl  ExtrapMethod=Clip  UseLastTableValue=on  InternalRulePriority=Speed  RndMeth=Simplest  InputSameDT=on
      settings: AttributesFormatString=|
      | %<Table>
      | %<BreakpointsForDimension1>
  1-D Lookup Table1 : Lookup_n-D  NumberOfTableDimensions=1  BreakpointsForDimension1=Mass_Props.propellant_bkpts  Table=Mass_Props.Ixy_tbl  ExtrapMethod=Clip  UseLastTableValue=on  InternalRulePriority=Speed  RndMeth=Simplest  InputSameDT=on
      settings: AttributesFormatString=|
      | %<Table>
      | %<BreakpointsForDimension1>
  1-D Lookup Table2 : Lookup_n-D  NumberOfTableDimensions=1  BreakpointsForDimension1=Mass_Props.propellant_bkpts  Table=Mass_Props.Ixz_tbl  ExtrapMethod=Clip  UseLastTableValue=on  InternalRulePriority=Speed  RndMeth=Simplest  InputSameDT=on
      settings: AttributesFormatString=|
      | %<Table>
      | %<BreakpointsForDimension1>
  1-D Lookup Table3 : Lookup_n-D  NumberOfTableDimensions=1  BreakpointsForDimension1=Mass_Props.propellant_bkpts  Table=Mass_Props.Iyx_tbl  ExtrapMethod=Clip  UseLastTableValue=on  InternalRulePriority=Speed  RndMeth=Simplest  InputSameDT=on
      settings: AttributesFormatString=|
      | %<Table>
      | %<BreakpointsForDimension1>
  1-D Lookup Table4 : Lookup_n-D  NumberOfTableDimensions=1  BreakpointsForDimension1=Mass_Props.propellant_bkpts  Table=Mass_Props.Iyy_tbl  ExtrapMethod=Clip  UseLastTableValue=on  InternalRulePriority=Speed  RndMeth=Simplest  InputSameDT=on
      settings: AttributesFormatString=|
      | %<Table>
      | %<BreakpointsForDimension1>
  1-D Lookup Table5 : Lookup_n-D  NumberOfTableDimensions=1  BreakpointsForDimension1=Mass_Props.propellant_bkpts  Table=Mass_Props.Iyz_tbl  ExtrapMethod=Clip  UseLastTableValue=on  InternalRulePriority=Speed  RndMeth=Simplest  InputSameDT=on
      settings: AttributesFormatString=|
      | %<Table>
      | %<BreakpointsForDimension1>
  1-D Lookup Table6 : Lookup_n-D  NumberOfTableDimensions=1  BreakpointsForDimension1=Mass_Props.propellant_bkpts  Table=Mass_Props.Izx_tbl  ExtrapMethod=Clip  UseLastTableValue=on  InternalRulePriority=Speed  RndMeth=Simplest  InputSameDT=on
      settings: AttributesFormatString=|
      | %<Table>
      | %<BreakpointsForDimension1>
  1-D Lookup Table7 : Lookup_n-D  NumberOfTableDimensions=1  BreakpointsForDimension1=Mass_Props.propellant_bkpts  Table=Mass_Props.Izy_tbl  ExtrapMethod=Clip  UseLastTableValue=on  InternalRulePriority=Speed  RndMeth=Simplest  InputSameDT=on
      settings: AttributesFormatString=|
      | %<Table>
      | %<BreakpointsForDimension1>
  1-D Lookup Table8 : Lookup_n-D  NumberOfTableDimensions=1  BreakpointsForDimension1=Mass_Props.propellant_bkpts  Table=Mass_Props.Izz_tbl  ExtrapMethod=Clip  UseLastTableValue=on  InternalRulePriority=Speed  RndMeth=Simplest  InputSameDT=on
      settings: AttributesFormatString=|
      | %<Table>
      | %<BreakpointsForDimension1>
  Add : Sum  Commented=on
  Add4 : Sum  Commented=on
  Add5 : Sum  Commented=on
  Constant15 : Constant  Commented=on  Value=JSPB_e
  JMMM_linear_interpolation : Subsystem  Commented=on
  Matrix Concatenate : Concatenate  NumInputs=3  Mode=Multidimensional array  ConcatenateDimension=2
  Terminator : Terminator  Commented=on
  Vector Concatenate : Concatenate  NumInputs=3
  Vector Concatenate1 : Concatenate  NumInputs=3
  Vector Concatenate2 : Concatenate  NumInputs=3
  mM D{1..9} (9 alike) : InportShadow  Port=2
  moi_coordinate_transformation : Subsystem  Commented=on
  moi_uncertainty : Subsystem
  steiners_theorem_missile : Subsystem  Commented=on
  steiners_theorem_motor : Subsystem  Commented=on
  JBBB : Outport  VectorParamsAs1DForOutWhenUnconnected=off
  wires:
  Matrix Concatenate/1 -> moi_uncertainty/1(JBBB_c)  "JBBB_c"
  [MOI_matrix_col3] -> Matrix Concatenate/3
  [MOI_matrix_col2] -> Matrix Concatenate/2
  [MOI_matrix_col1] -> Matrix Concatenate/1
  Vector Concatenate2/1 -> [MOI_matrix_col3]
  Vector Concatenate1/1 -> [MOI_matrix_col2]
  Vector Concatenate/1 -> [MOI_matrix_col1]
  1-D Lookup Table8/1 -> Vector Concatenate2/3
  1-D Lookup Table5/1 -> Vector Concatenate2/2
  1-D Lookup Table2/1 -> Vector Concatenate2/1
  1-D Lookup Table7/1 -> Vector Concatenate1/3
  1-D Lookup Table4/1 -> Vector Concatenate1/2
  1-D Lookup Table1/1 -> Vector Concatenate1/1
  1-D Lookup Table/1 -> Vector Concatenate/1
  1-D Lookup Table3/1 -> Vector Concatenate/2
  1-D Lookup Table6/1 -> Vector Concatenate/3
  mM D9/1 -> 1-D Lookup Table8/1
  mM D8/1 -> 1-D Lookup Table5/1
  mM D7/1 -> 1-D Lookup Table2/1
  mM D6/1 -> 1-D Lookup Table7/1
  mM D5/1 -> 1-D Lookup Table4/1
  mM D4/1 -> 1-D Lookup Table1/1
  mM D3/1 -> 1-D Lookup Table6/1
  mM D2/1 -> 1-D Lookup Table3/1
  mM D1/1 -> 1-D Lookup Table/1
  moi_uncertainty/1(JBBB) -> JBBB/1
  Add4/1 -> Terminator/1  "JBBB_c"
  steiners_theorem_missile/1(J_deviation) -> Add5/2
  Add5/1 -> Add4/1  "JSBB"
  Constant15/1 -> Add5/1
  Add/1 -> Add4/2  "JMBB"
  steiners_theorem_motor/1(JM_deviation) -> Add/1
  pBPB/1 -> steiners_theorem_motor/1(pBPB), steiners_theorem_missile/1(pBPB)
  moi_coordinate_transformation/1(JMMB) -> Add/2
  JMMM_linear_interpolation/1(JMMM) -> moi_coordinate_transformation/1(JMMM)
  mM/1 -> JMMM_linear_interpolation/1(mM), steiners_theorem_motor/2(mM)

== system PIL_NO_RPI/Non-linear Flight Dynamic Model2/environment_global/atm_dynamic/trafo_around_z_axis ==
  vec1 : Inport
  gamma : Inport  Port=2
  1_rot_mat : Subsystem  mask(Rotation um 1, 2 oder 3 Achsen){rot_1=Rotation um z-Achse}
      mask prompts: rot_1 "1. Rotation"
      mask help:
      | Dieser Block liefert die Rotationsmatrix T12 für den Fall zurück, dass sich das Ziel-Koordinatensystem (1) durch Drehungen um 1, 2 oder 3 Achsen gegenüber dem Ausgangskoordinatensystem (2) beschreiben lässt (passive Drehung).
      |
      | Die Anzahl der Rotation sowie die Reihenfolge ist frei einstellbar.
      |
      | Die Rotationswinkel haben die Einheit [rad].
      mask TypeOptions rot_1: Rotation um x-Achse | Rotation um y-Achse | Rotation um z-Achse
  Product : Product  Multiplication=Matrix(*)
  Reshape : Reshape  OutputDimensionality=Column vector (2-D)
  vec2 : Outport  VectorParamsAs1DForOutWhenUnconnected=off
  wires:
  Product/1 -> vec2/1  "vec2"
  gamma/1 -> 1_rot_mat/1(wi1)  "gamma"
  1_rot_mat/1(T12) -> Product/1  "T12"
  vec1/1 -> Reshape/1  "vec1"
  Reshape/1 -> Product/2  "vec1"

== system PIL_NO_RPI/Flight Control Computer/Pixhawk1/FCC Logic1/Control/Phi Controller ==
  phi_cmd_rad : Inport
  phi_rad : Inport  Port=2
  p_rps : Inport  Port=3
  Reset Integrators : Inport  Port=4
  V_mps : Inport  Port=5
  h_m : Inport  Port=6
  Trigger : TriggerPort  VariantControl=Variant  PortDimensions=1
  Bus Selector : BusSelector  OutputSignals=Kp_p,Ki_phi,Kp_phi
  Constant : Constant  Value=0  OutDataTypeStr=single
  Discrete-Time Integrator : DiscreteIntegrator  ExternalReset=level  InitialConditionSource=external  SampleTime=-1  OutDataTypeStr=single  ICPrevOutput=DiscIntNeverNeededParam  ICPrevScaledInput=DiscIntNeverNeededParam
  Gain_Lookup : Subsystem
  Product1 : Product
  Product2 : Product
  Product3 : Product
  Sum3 : Sum  Inputs=|+-
  Sum4 : Sum  Inputs=++|
  Sum5 : Sum  Inputs=|+-
  dela_cmd_rad : Outport
  wires:
  Gain_Lookup/1(Gains) -> Bus Selector/1
  Bus Selector/2 -> [Ki_phi]  "<Ki_phi>"
  Product1/1 -> dela_cmd_rad/1
  Bus Selector/3 -> [Kp_phi]  "<Kp_phi>"
  phi_cmd_rad/1 -> Sum3/1
  [Kp_phi] -> Product2/1
  h_m/1 -> Gain_Lookup/2(h_m)
  Sum4/1 -> Sum5/1
  Reset Integrators/1 -> Discrete-Time Integrator/2
  p_rps/1 -> Sum5/2
  Product3/1 -> Discrete-Time Integrator/1
  [Kp_p] -> Product1/1
  [Ki_phi] -> Product3/1
  Sum5/1 -> Product1/2
  Discrete-Time Integrator/1 -> Sum4/2  "phi_int"
  V_mps/1 -> Gain_Lookup/1(V_mps)
  Constant/1 -> Discrete-Time Integrator/3
  Sum3/1 -> Product3/2, Product2/2
  Product2/1 -> Sum4/1
  phi_rad/1 -> Sum3/2
  Bus Selector/1 -> [Kp_p]  "<Kp_p>"

== system PIL_NO_RPI/Flight Control Computer/Pixhawk1/FCC Logic1/Control/Subsystem ==
  <u> : Inport
  <v> : Inport  Port=2
  <w> : Inport  Port=3
  Add : Sum  Inputs=+++
  Square : Math  Operator=square  SaturateOnIntegerOverflow=on
  Square Root : Sqrt  SaturateOnIntegerOverflow=on
  Square1 : Math  Operator=square  SaturateOnIntegerOverflow=on
  Square2 : Math  Operator=square  SaturateOnIntegerOverflow=on
  U : Outport
  wires:
  Square2/1 -> Add/3
  Square Root/1 -> U/1
  Add/1 -> Square Root/1
  Square1/1 -> Add/2
  <u>/1 -> Square/1
  Square/1 -> Add/1
  <v>/1 -> Square1/1
  <w>/1 -> Square2/1

== system PIL_NO_RPI/Flight Control Computer/Pixhawk1/FCC Logic1/Fin Allocation1/control_allocation ==
  fin_cmd : Inport
  Constant7 : Constant  Value=HIL_Data.FDM.Tr4r3  OutDataTypeStr=single
  Product : Product  Multiplication=Matrix(*)
  siB_cmd : Outport  VectorParamsAs1DForOutWhenUnconnected=off
  wires:
  Constant7/1 -> Product/1
  fin_cmd/1 -> Product/2
  Product/1 -> siB_cmd/1  "siB_cmd"

== system PIL_NO_RPI/Flight Control Computer/Pixhawk1/FCC Logic1/Fin Allocation2/Subsystem ==
  fin_cmd : Inport
  Demux : Demux
  Vector Concatenate : Concatenate  NumInputs=4
  control_allocation : Subsystem
  siB_cmd : Outport
  wires:
  Demux/2 -> Vector Concatenate/2  "siB_cmd_2"
  control_allocation/1(siB_cmd) -> Demux/1
  Vector Concatenate/1 -> siB_cmd/1  "siB_cmd"
  Demux/3 -> Vector Concatenate/3  "siB_cmd_3"
  Demux/1 -> Vector Concatenate/1  "siB_cmd_1"
  Demux/4 -> Vector Concatenate/4  "siB_cmd_4"
  fin_cmd/1 -> control_allocation/1(fin_cmd)

== system PIL_NO_RPI/Non-linear Flight Dynamic Model1/Environment/atm_dynamic/trafo_around_z_axis/1_rot_mat ==
  wi1 : Inport
  1. Rotation x-Achse : Subsystem
  1. Rotation y-Achse : Subsystem
  1. Rotation z-Achse : Subsystem
  Constant : Constant  Value=rot_1
  Multiport Switch : MultiPortSwitch
  T12 : Outport  VectorParamsAs1DForOutWhenUnconnected=off
  wires:
  Constant/1 -> Multiport Switch/1
  1. Rotation x-Achse/1(1Rot_Matrix_x) -> Multiport Switch/2
  1. Rotation y-Achse/1(1Rot_Matrix_y) -> Multiport Switch/3
  1. Rotation z-Achse/1(1Rot_Matrix_z) -> Multiport Switch/4
  wi1/1 -> 1. Rotation x-Achse/1(alpha1), 1. Rotation z-Achse/1(alpha1), 1. Rotation y-Achse/1(alpha1)
  Multiport Switch/1 -> T12/1  "T12"

== system PIL_NO_RPI/Non-linear Flight Dynamic Model1/Extract States/Assemble_States_Bus1/Three-axis Inertial Measurement Unit3/Acceleration Conversion ==
  acceleration : Inport  Unit=m/s^2
  Unit Conversion : UnitConversion
  inherit : Outport  VectorParamsAs1DForOutWhenUnconnected=off
  wires:
  acceleration/1 -> Unit Conversion/1
  Unit Conversion/1 -> inherit/1
